simulink model "sedemo_videoframeprocessing"  (Simulink 7.5)
settings: Solver=VariableStepDiscrete  StartTime=0.0  StopTime=20  MaxStep=inf  RelTol=1e-3
undefined symbols (not defined in the file or in its folder): des_figposition
libraries: simeventssink1 x5, simeventsrouting1 x3, simeventsqueue1 x2, simeventsserver1 x2, simeventsgenerators1 x2, simeventsattributes2 x2, simeventsinfo x1
settings Model: Creator=The MathWorks Inc.  ExtModeAutoUpdateStatusClock=off
settings DataIOCC: SaveOutput=off  SaveTime=off
settings OptimizationCC: InitFltsAndDblsToZero=on
settings DebuggingCC: AlgebraicLoopMsg=error  SignalResolutionControl=TryResolveAllWithWarning  SolverPrmCheckMsg=none  StrictBusMsg=Warning
settings SimEventsCC: propDiagAttribOutput=1  propDiagFcnCallOutput=1  propDiagStatOutput=0

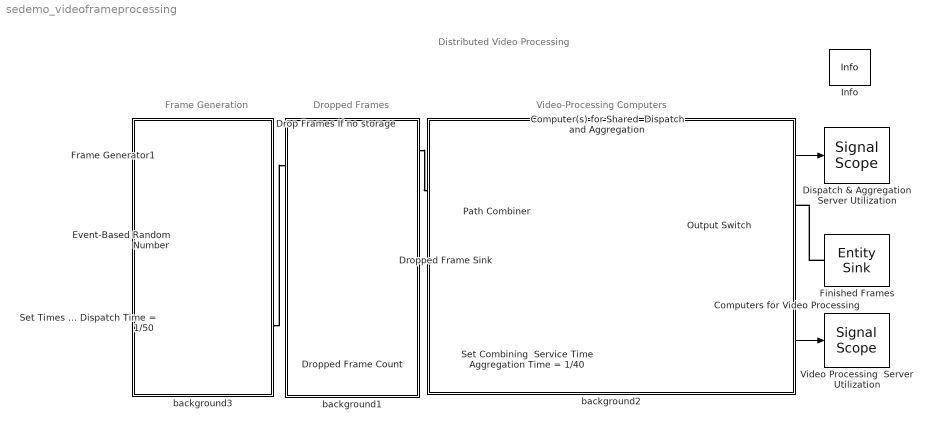
== system sedemo_videoframeprocessing ==
  note: Distributed Video Processing
  note: Dropped Frames
  note: Video-Processing Computers
  note: Frame Generation
  "Computer(s) for Shared  Dispatch and Aggregation " : Subsystem  mask(Buffered Servers){NumServers=1}
      mask prompts: NumServers "Number of Servers"
      mask help: Dispatch Queue and N-Blade Server pair in which the Dispatch Queue block capacity is the same as the number of servers in the N- Blade Server block capacity.
      settings: AttributesFormatString=Num. Servers = %<NumServers>
      mask Display: text(20,30,'Buffered\nServer(s)')
  "Computers for Video Processing " : Subsystem  mask(Buffered Servers){NumServers=5}
      mask prompts: NumServers "Number of Servers"
      mask help: Dispatch Queue and N-Blade Server pair in which the Dispatch Queue block capacity is the same as the number of servers in the N- Blade Server block capacity.
      settings: AttributesFormatString=Num. Servers = %<NumServers>
      mask Display: text(20,30,'   Buffered\n   Servers')
  Dispatch & Aggregation Server Utilization : simeventssink1/Signal Scope  Priority=1  SystemSampleTime=-1  PlotType=Continuous  InputType=Signal  NumInputs=1  AttributeNameY=Count  XInputOptionSignal=Event time  XInputOptionEntity=Event time  AttributeNameX=Count  EnableEntityOutport=on  XMin=0  XMax=10  XLimitExceededOption=Stretch axis limits  YLimitExceededOption=Stretch axis limits  AxisGrid=on  AxisLegend=off  LineDisables=""  LineColors=b  LineStyles=-  LineMarkers=None  OpenScopeAtSimStart=on  Title=Dispatching and Combining Utilization  YLabel=CPU Utilization  XLabel=Time  FigurePosition=des_figposition([75 72 25 22])  AxisZoom=off  DataStoreOption=Limited  DataPointsLimit=10000  StatNumberArrived=Off  ShowCountPlotted=off  ShowToolbar=off
      settings: YMin=0  YMax=1
  Drop Frames If no storage : simeventsrouting1/Output Switch  Priority=1  SystemSampleTime=-1  NumberOutputPorts=2  SwitchingCriterion=First port that is not blocked  InitialSeed=34567  AttributeName=Attribute1  InitialConditionsOpt=off  InitialConditions=1  EntityBufferOpt=off  SpecifyEventPriority=off  PriorityOutputSwitchSelectPort=4100  TimeoutPortOpt=off  StatNumberDeparted=Off  StatNumberTimedOut=Off  StatPendingEntity=Off  StatLastDeparturePort=Off  EvaluatedNumPorts=2
  Dropped Frame Count : simeventssink1/Signal Scope  Priority=1  SystemSampleTime=-1  PlotType=Stair  InputType=Signal  NumInputs=1  AttributeNameY=Count  XInputOptionSignal=Event time  XInputOptionEntity=Event time  AttributeNameX=Count  EnableEntityOutport=on  XMin=0  XMax=20  XLimitExceededOption=Stretch axis limits  YLimitExceededOption=Stretch axis limits  AxisGrid=on  AxisLegend=off  LineDisables=""  LineColors=b  LineStyles=-  LineMarkers=.  OpenScopeAtSimStart=on  Title=Count of Dropped Frames  YLabel=Dropped Frames  XLabel=Time  FigurePosition=des_figposition([5 10 25 22])  AxisZoom=off  DataStoreOption=Limited  DataPointsLimit=10000  StatNumberArrived=Off  ShowCountPlotted=off  ShowToolbar=off
      settings: YMin=0  YMax=10
  Dropped Frame Sink : simeventssink1/Entity Sink  Priority=1  SystemSampleTime=-1  AvailableForArrivals=on  StatNumberArrived=On
  Event-Based Random Number : simeventsgenerators1/Signal Generators/Event-Based Random Number  SystemSampleTime=-1  distribution=Uniform  meanExp=1/10  minUnif=1/8  maxUnif=1/5  pOneBern=0.25  pSuccessBino=0.5  numTrialBino=1  meanNorm=0  stdNorm=1  minTri=1  maxTri=3  modeTri=2  thresholdLogn=0  scaleLogn=1  shapeLogn=1  pSuccessGeo=0.5  meanPoiss=1  thresholdLogl=0  scaleLogl=1  thresholdGam=0  scaleGam=1  shapeGam=1  minBeta=0  maxBeta=1  shape1Beta=1  shape2Beta=1  minUnid=0  maxUnid=1  numValueUnid=2  thresholdWbl=0  scaleWbl=1  shapeWbl=1  valueVecCont=[0 1]  cdfVecCont=[0 1]  valueVecDisc=[0 1]  probVecDisc=[0.5 0.5]  seed=12345  IsProcessed=on  isConnected=1
  Finished Frames : simeventssink1/Entity Sink  Priority=1  SystemSampleTime=-1  AvailableForArrivals=on  StatNumberArrived=Off
  Frame Generator1 : simeventsgenerators1/Entity Generators/Time-Based Entity Generator  Priority=1  DialogController=des_ddg_create  DialogControllerArgs=DataTag10  SystemSampleTime=-1  GenerateEntitiesUpon=Intergeneration time from dialog  Distribution=Constant  Minimum=0  Maximum=1  Mean=1  InitialSeed=12345  Period=1/30  PriorityEntityGeneration=300  GenerateEntityAtSimulationStart=on  ResponseWhenBlocked=Pause generation  ResponseWhenUnblocked=Immediate restart  EntityType=Standard  StatNumberDeparted=Off  StatPendingEntity=Off  StatAverageIntergenerationTime=Off
      settings: AttributesFormatString=Period = %<Period>
  Info : simeventsinfo/Info  SystemSampleTime=-1
  Output Switch : simeventsrouting1/Output Switch  Priority=1  SystemSampleTime=-1  NumberOutputPorts=2  SwitchingCriterion=From attribute  InitialSeed=34567  AttributeName=IsDoneFlag  InitialConditionsOpt=off  InitialConditions=1  EntityBufferOpt=off  SpecifyEventPriority=off  PriorityOutputSwitchSelectPort=4100  TimeoutPortOpt=off  StatNumberDeparted=Off  StatNumberTimedOut=Off  StatPendingEntity=Off  StatLastDeparturePort=Off  EvaluatedNumPorts=2
  Path Combiner : simeventsrouting1/Path Combiner  Priority=1  SystemSampleTime=-1  NumberInputPorts=2  InputPortPrecedence=IN1 port  InitialSeed=45675  SpecifyEventPriority=off  PriorityPathCombinerPortPrecedenceSelection=4100  StatNumberDeparted=Off  StatLastArrivalPort=Off  EvaluatedNumPorts=2
  Set Combining  Service Time Aggregation Time = 1/40 : simeventsattributes2/Set Attribute  Priority=1  DialogController=des_ddg_create  DialogControllerArgs=DataTag14  SystemSampleTime=-1  AttributeFrom=Dialog|Dialog  AttributeName=IsDoneFlag|DispCombServiceTime  AttributeTreatAsVector=1|1  AttributeValue=2|1/40  AttributeCreate=on  StatNumberDeparted=Off  EvaluatedAttributeValue={2;1/40}
  Set Times ... Dispatch Time = 1/50 : simeventsattributes2/Set Attribute  Priority=1  DialogController=des_ddg_create  DialogControllerArgs=DataTag16  SystemSampleTime=-1  AttributeFrom=Dialog|Dialog|Signal port  AttributeName=IsDoneFlag|DispCombServiceTime|BladeServiceTime  AttributeTreatAsVector=1|1|1  AttributeValue=1|1/50|1  AttributeCreate=on  StatNumberDeparted=Off  EvaluatedAttributeValue={1;1/50;[]}
  Video Processing  Server Utilization : simeventssink1/Signal Scope  Priority=1  SystemSampleTime=-1  PlotType=Continuous  InputType=Signal  NumInputs=1  AttributeNameY=Count  XInputOptionSignal=Event time  XInputOptionEntity=Event time  AttributeNameX=Count  EnableEntityOutport=on  XMin=0  XMax=10  XLimitExceededOption=Stretch axis limits  YLimitExceededOption=Stretch axis limits  AxisGrid=on  AxisLegend=off  LineDisables=""  LineColors=b  LineStyles=-  LineMarkers=None  OpenScopeAtSimStart=on  Title=Video Processing Utilization  YLabel=CPU Utilization  XLabel=Time  FigurePosition=des_figposition([75 40 25 22])  AxisZoom=off  DataStoreOption=Limited  DataPointsLimit=10000  StatNumberArrived=Off  ShowCountPlotted=off  ShowToolbar=off
      settings: YMin=0  YMax=1
  background1 : Subsystem
      mask Display: disp('')
  background2 : Subsystem
      mask Display: disp('')
  background3 : Subsystem
      mask Display: disp('')
  wires:
  Dropped Frame Sink/1 -> Dropped Frame Count/1
  "Computers for Video Processing "/1(util) -> Video Processing  Server Utilization/1
  "Computer(s) for Shared  Dispatch and Aggregation "/1(util) -> Dispatch & Aggregation Server Utilization/1
  Event-Based Random Number/1 -> Set Times ... Dispatch Time = 1/50/1
  connections:
  Drop Frames If no storage/RConn2 -- Dropped Frame Sink/LConn1
  Drop Frames If no storage/RConn1 -- Path Combiner/LConn2
  Set Combining  Service Time Aggregation Time = 1/40/RConn1 -- Path Combiner/LConn1
  Finished Frames/LConn1 -- Output Switch/RConn2
  Set Combining  Service Time Aggregation Time = 1/40/LConn1 -- "Computers for Video Processing "/RConn1
  Output Switch/RConn1 -- "Computers for Video Processing "/LConn1
  Path Combiner/RConn1 -- "Computer(s) for Shared  Dispatch and Aggregation "/LConn1
  "Computer(s) for Shared  Dispatch and Aggregation "/RConn1 -- Output Switch/LConn1
  Frame Generator1/RConn1 -- Set Times ... Dispatch Time = 1/50/LConn1
  Set Times ... Dispatch Time = 1/50/RConn1 -- Drop Frames If no storage/LConn1

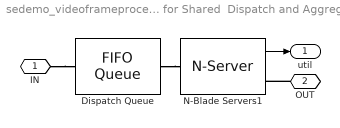
== system sedemo_videoframeprocessing/Computer(s) for Shared  Dispatch and Aggregation  ==
  Dispatch Queue : simeventsqueue1/FIFO Queue  Priority=1  SystemSampleTime=-1  Capacity=NumServers  EnableTOPort=off  StatNumberDeparted=Off  StatNumberInBlock=Off  StatPendingEntity=Off  StatAverageWait=Off  StatAverageQueueLength=Off  StatNumberTimedout=Off
  N-Blade Servers1 : simeventsserver1/N-Server  Priority=1  SystemSampleTime=-1  NumberOfServers=NumServers  ServiceTimeFrom=Attribute  ServiceTime=1  AttributeName=DispCombServiceTime  PriorityServiceCompletion=450  EnableTOPort=off  StatNumberDeparted=Off  StatNumberInBlock=Off  StatPendingEntity=Off  StatNumberPending=Off  StatAverageWait=Off  StatUtilization=On  StatNumberTimedout=Off
  IN : PMIOPort  Port=1  Side=Left
  OUT : PMIOPort  Port=2  Side=Right
  util : Outport  OutDataType=sfix(16)  OutScaling=2^0
  wires:
  N-Blade Servers1/1 -> util/1
  connections:
  Dispatch Queue/RConn1 -- N-Blade Servers1/LConn1
  IN/RConn1 -- Dispatch Queue/LConn1
  OUT/RConn1 -- N-Blade Servers1/RConn1

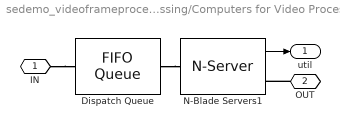
== system sedemo_videoframeprocessing/Computers for Video Processing  ==
  Dispatch Queue : simeventsqueue1/FIFO Queue  Priority=1  SystemSampleTime=-1  Capacity=NumServers  EnableTOPort=off  StatNumberDeparted=Off  StatNumberInBlock=Off  StatPendingEntity=Off  StatAverageWait=Off  StatAverageQueueLength=Off  StatNumberTimedout=Off
  N-Blade Servers1 : simeventsserver1/N-Server  Priority=1  SystemSampleTime=-1  NumberOfServers=NumServers  ServiceTimeFrom=Attribute  ServiceTime=1  AttributeName=BladeServiceTime  PriorityServiceCompletion=450  EnableTOPort=off  StatNumberDeparted=Off  StatNumberInBlock=Off  StatPendingEntity=Off  StatNumberPending=Off  StatAverageWait=Off  StatUtilization=On  StatNumberTimedout=Off
  IN : PMIOPort  Port=1  Side=Left
  OUT : PMIOPort  Port=2  Side=Right
  util : Outport  OutDataType=sfix(16)  OutScaling=2^0
  wires:
  N-Blade Servers1/1 -> util/1
  connections:
  Dispatch Queue/RConn1 -- N-Blade Servers1/LConn1
  IN/RConn1 -- Dispatch Queue/LConn1
  OUT/RConn1 -- N-Blade Servers1/RConn1

== system sedemo_videoframeprocessing/background1 ==

== system sedemo_videoframeprocessing/background2 ==

== system sedemo_videoframeprocessing/background3 ==
